simulink model "AM_Communication_System"  (Simulink 8.7)
settings: Solver=VariableStepAuto  StartTime=0.0  StopTime=1  RelTol=1e-3
libraries: commchan3 x1, dspfdesign x1
settings Model: Creator=tp033402  LastModifiedBy=Muhammad Zubair
settings DataIOCC: SignalLoggingSaveFormat=ModelDataLogs
settings OptimizationCC: ExpressionDepthLimit=2147483647
settings DebuggingCC: SolverPrmCheckMsg=warning  FcnCallInpInsideContextMsg=UseLocalSettings  StateNameClashWarn=warning
settings GRTTargetCC: CombineOutputUpdateFcns=off  GRTInterface=on

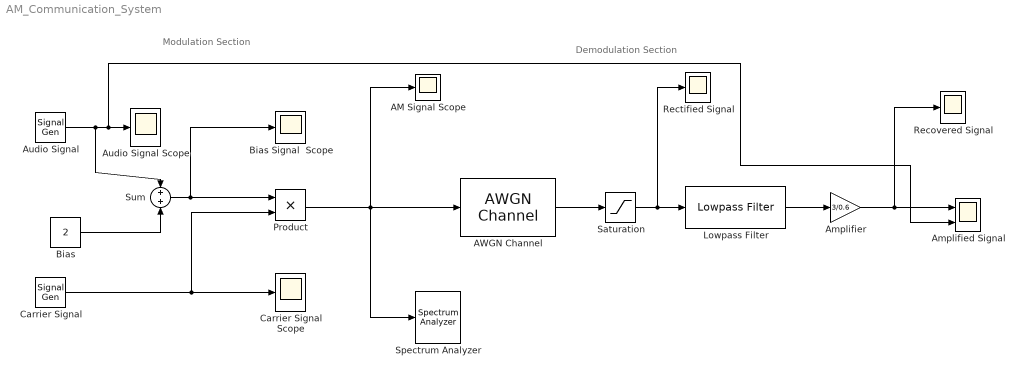
== system AM_Communication_System ==
  note: Modulation Section
  note: Demodulation Section
  AM Signal Scope : Scope
  AWGN Channel : commchan3/AWGN Channel  InputProcessing=Columns as channels (frame based)  seed=67  noiseMode="Signal to noise ratio  (SNR)"  EbNodB=10  EsNodB=10  SNRdB=10  bitsPerSym=1  Ps=1  Tsym=1  variance=1
  Amplified Signal : Scope  NumInputPorts=2
  Amplifier : Gain  Gain=3/0.6
  Audio Signal : SignalGenerator  Amplitude=0.8  Frequency=10
  Audio Signal Scope : Scope
  Bias : Constant  Value=2
  Bias Signal  Scope : Scope
  Carrier Signal : SignalGenerator  Amplitude=2  Frequency=100
  Carrier Signal Scope : Scope
  Lowpass Filter : dspfdesign/Lowpass Filter  FilterType=FIR  DesignForMinimumOrder=on  FilterOrder=50  PassbandFrequency=2*pi*10  StopbandFrequency=2*pi*110  PassbandRipple=0.1  StopbandAttenuation=80  InheritSampleRate=off  SampleRate=44100  roundingMode=Floor  coeffsDataTypeStr=fixdt(1,16)  SimulateUsing=Interpreted execution
  Product : Product  SampleTime=0.001  RndMeth=Zero
  Recovered Signal : Scope
  Rectified Signal : Scope
  Saturation : Saturate  UpperLimit=8  LowerLimit=0
  Spectrum Analyzer : SpectrumAnalyzer
  Sum : Sum  Inputs=2  SampleTime=0.001
  wires:
  Bias/1 -> Sum/2
  Sum/1 -> Product/1, Bias Signal  Scope/1
  Carrier Signal/1 -> Carrier Signal Scope/1, Product/2
  Audio Signal/1 -> Sum/1, Amplified Signal/2, Audio Signal Scope/1
  Saturation/1 -> Lowpass Filter/1, Rectified Signal/1
  AWGN Channel/1 -> Saturation/1
  Product/1 -> Spectrum Analyzer/1, AWGN Channel/1, AM Signal Scope/1
  Lowpass Filter/1 -> Amplifier/1
  Amplifier/1 -> Recovered Signal/1, Amplified Signal/1
